simulink model "sgMdl_ModbusRTU_1CLI3SRV"  (R2024b)
settings: Solver=FixedStepAuto  StartTime=0.0  StopTime=inf  RelTol=1e-3  EnableMultiTasking=on
undefined symbols (not defined in the file): standard
libraries: speedgoatlib_mbrtu x14, slrealtimeutilitieslib x10, speedgoatlib_serial x1
Description:
  | Modbus RTU Multi-Node Loopback
settings Model: sg_rtwmakecfg_data=_sg_IO75X_v1_2_0__sg_netxLib_MSVC140_  ModifiedByFormat=Speedgoat  SimulationMode=external  ExtModeTrigDuration=100000  Creator=Speedgoat  LastModifiedBy=Speedgoat
settings SolverCC: ConcurrentTasks=on  AlgebraicLoopSolver=TrustRegion  PositivePriorityOrder=on  AutoInsertRateTranBlk=on  InsertRTBMode=Never (minimum delay)
settings DataIOCC: LimitDataPoints=on  SaveFormat=StructureWithTime  ReturnWorkspaceOutputs=off
settings OptimizationCC: BlockReduction=off  BooleanDataType=off  OptimizeBlockIOStorage=off  BufferReuse=off  GlobalBufferReuse=off  ExpressionFolding=off  LocalBlockOutputs=off  OptimizeDataStoreBuffers=off  BusAssignmentInplaceUpdate=off
settings DebuggingCC: SaveWithParameterizedLinksMsg=none  UnderspecifiedInitializationDetection=Classic  MergeDetectMultiDrivingBlocksExec=none  SignalResolutionControl=TryResolveAllWithWarning  InheritedTsInSrcMsg=none  TasksWithSamePriorityMsg=none  ParameterOverflowMsg=warning  UnconnectedInputMsg=warning  UnconnectedOutputMsg=warning  UnconnectedLineMsg=warning  SFUnexpectedBacktrackingDiag=warning  SFNoUnconditionalDefaultTransitionDiag=warning  SFExecutionAtInitializationDiag=none  ArithmeticOperatorsInVariantConditions=warning
settings HardwareCC: ProdBitPerLong=64  ProdLongLongMode=on  ProdHWDeviceType=Intel->x86-64 (Linux 64)  TargetBitPerPointer=64  TargetBitPerSizeT=64  TargetBitPerPtrDiffT=64  TargetLongLongMode=on  TargetIntDivRoundTo=Zero  TargetEndianess=LittleEndian  TargetWordSize=64  TargetHWDeviceType=MATLAB Host
settings ModelReferenceCC: EnableRefExpFcnMdlSchedulingChecks=on  PropagateSignalLabelsOutOfModel=off
settings SFSimCC: SimUseLocalCustomCode=off  CustomCodeUndefinedFunction=UseInterfaceOnly
settings RTWCC: Description=Speedgoat Real-Time Target Machine  SystemTargetFile=speedgoat.tlc  TemplateMakefile=slrealtime_default_tmf  RetainRTWFile=on  RTWUseLocalCustomCode=off  Toolchain=Simulink Real-Time Toolchain  BuildConfiguration=Faster Runs  TargetLang=C++  GPUComputeCapability=3.5  DLArmComputeVersion=19.05
settings CodeAppCC: StateflowObjectComments=on
settings SimulinkRealTimeTargetCC: SubcomponentCodeInterfacePackaging=Reusable function  InstructionSetFMA=off  LogToMDFFile=off  SLRTFileLogMaxRuns=10
settings ConfigComp: CovMetricSettings=dw  CovSaveCumulativeToWorkspaceVar=on  CovSaveSingleToWorkspaceVar=on  CovExternalEMLEnable=off  CovBoundaryAbsTol=1.0e-5

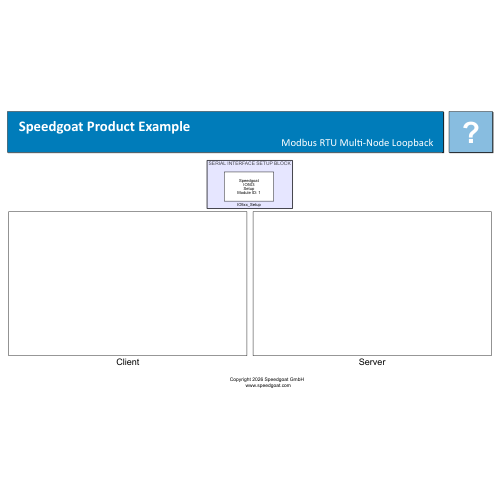
[thumbnail: Simulink's stored preview of the top-level diagram]
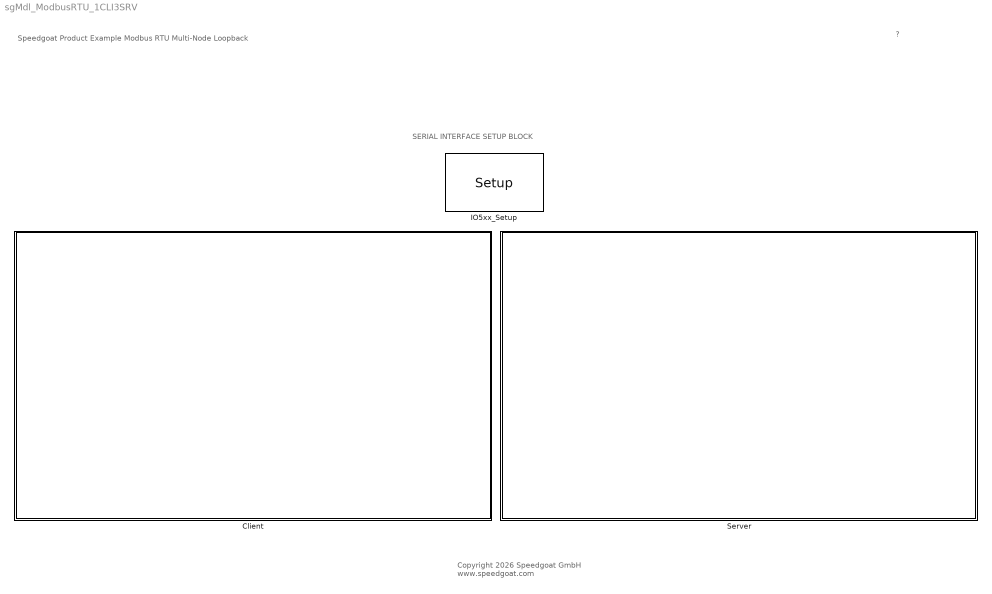
== system sgMdl_ModbusRTU_1CLI3SRV ==
  note: SERIAL INTERFACE SETUP BLOCK
  note: Speedgoat Product Example
      | Modbus RTU Multi-Node Loopback
  note: ?
  note: Copyright 2026 Speedgoat GmbH
      |  www.speedgoat.com
  Client : Subsystem
  IO5xx_Setup : speedgoatlib_serial/Speedgoat Shared blocks/Setup   parModuleType=IO504  parModuleId=1  parSlot=-1  parOscillator=50  parOscillator581=125  parTransceiver1=RS485 Half-Duplex  parTransceiver2=Disabled  parTransceiver3=RS485 Half-Duplex  parTransceiver4=Disabled  parTransceiver5=Disabled  parTransceiver6=Disabled  parTransceiver7=Disabled  parTransceiver8=Disabled  parTxTerm1=on  parRxTerm1=off  parMessageMonitoring1=off  parAutoTurnaround1=off  parTurnaroundDelay1=0  parStandardBaud1=off  parBaudrate1=19200  parBaudDivisor1=25  parSamplingRate1=16x (standard)  parPrescale1=4x  parCalcBaud1=31250  parParity1=Even  parDataBits1=8  parStopBits1=1  parTxTrigLvl1=1  parRxTrigLvl1=56  parHandshake1=none  parRtsHysteresis1=0  parXon1=17  parXoff1=19  parTxSwFifoSize1=1024  parRxSwFifoSize1=1024  parTxTerm2=on  parRxTerm2=off  parMessageMonitoring2=off  parAutoTurnaround2=off  parTurnaroundDelay2=0  parStandardBaud2=off  parBaudrate2=19200  parBaudDivisor2=1  parSamplingRate2=16x (standard)  parPrescale2=None  parCalcBaud2=3125000  parParity2=Even  parDataBits2=8  parStopBits2=1  parTxTrigLvl2=1  parRxTrigLvl2=56  parHandshake2=none  parRtsHysteresis2=0  parXon2=17  parXoff2=19  parTxSwFifoSize2=1024  parRxSwFifoSize2=1024  parTxTerm3=on  parRxTerm3=off  parMessageMonitoring3=off  parAutoTurnaround3=off  parTurnaroundDelay3=0  parStandardBaud3=off  parBaudrate3=19200  parBaudDivisor3=25  parSamplingRate3=16x (standard)  parPrescale3=4x  parCalcBaud3=31250  parParity3=Even  parDataBits3=8  parStopBits3=1  parTxTrigLvl3=1  parRxTrigLvl3=56  parHandshake3=none  parRtsHysteresis3=0  parXon3=17  parXoff3=19  parTxSwFifoSize3=1024  parRxSwFifoSize3=1024  parTxTerm4=off  parRxTerm4=off  parMessageMonitoring4=off  parAutoTurnaround4=off  parTurnaroundDelay4=0  parStandardBaud4=off  parBaudrate4=921600  parBaudDivisor4=1  parSamplingRate4=16x (standard)  parPrescale4=None  parCalcBaud4=3125000  parParity4=None  parDataBits4=8  parStopBits4=1  parTxTrigLvl4=1  parRxTrigLvl4=1  parHandshake4=none  parRtsHysteresis4=0  parXon4=17  parXoff4=19  parTxSwFifoSize4=1024  parRxSwFifoSize4=1024  parTxTerm5=off  parRxTerm5=off  parMessageMonitoring5=off  parAutoTurnaround5=off  parTurnaroundDelay5=0  parStandardBaud5=off  parBaudrate5=921600  parBaudDivisor5=1  parSamplingRate5=16x (standard)  parPrescale5=None  parCalcBaud5=3125000  parParity5=None  parDataBits5=8  parStopBits5=1  parTxTrigLvl5=1  parRxTrigLvl5=1  parHandshake5=none  parRtsHysteresis5=0  parXon5=17  parXoff5=19  parTxSwFifoSize5=1024  parRxSwFifoSize5=1024  parTxTerm6=on  parRxTerm6=off  parMessageMonitoring6=off  parAutoTurnaround6=off  parTurnaroundDelay6=0  parStandardBaud6=off  parBaudrate6=921600  parBaudDivisor6=1  parSamplingRate6=16x (standard)  parPrescale6=None  parCalcBaud6=3125000  parParity6=None  parDataBits6=8  parStopBits6=1  parTxTrigLvl6=1  parRxTrigLvl6=1  parHandshake6=none  parRtsHysteresis6=0  parXon6=17  parXoff6=19  parTxSwFifoSize6=1024  parRxSwFifoSize6=1024  parTxTerm7=off  parRxTerm7=off  parMessageMonitoring7=off  parAutoTurnaround7=off  parTurnaroundDelay7=0  parStandardBaud7=off  parBaudrate7=921600  parBaudDivisor7=1  parSamplingRate7=16x (standard)  parPrescale7=None  parCalcBaud7=3125000  parParity7=None  parDataBits7=8  parStopBits7=1  parTxTrigLvl7=1  parRxTrigLvl7=1  parHandshake7=none  parRtsHysteresis7=0  parXon7=17  parXoff7=19  parTxSwFifoSize7=1024  parRxSwFifoSize7=1024  parTxTerm8=off  parRxTerm8=off  parMessageMonitoring8=off  parAutoTurnaround8=off  parTurnaroundDelay8=0  parStandardBaud8=off  parBaudrate8=921600  parBaudDivisor8=1  parSamplingRate8=16x (standard)  parPrescale8=None  parCalcBaud8=3125000  parParity8=None  parDataBits8=8  parStopBits8=1  parTxTrigLvl8=1  parRxTrigLvl8=1  parHandshake8=none  parRtsHysteresis8=0  parXon8=17  parXoff8=19  parTxSwFifoSize8=1024  parRxSwFifoSize8=1024
  Server : Subsystem

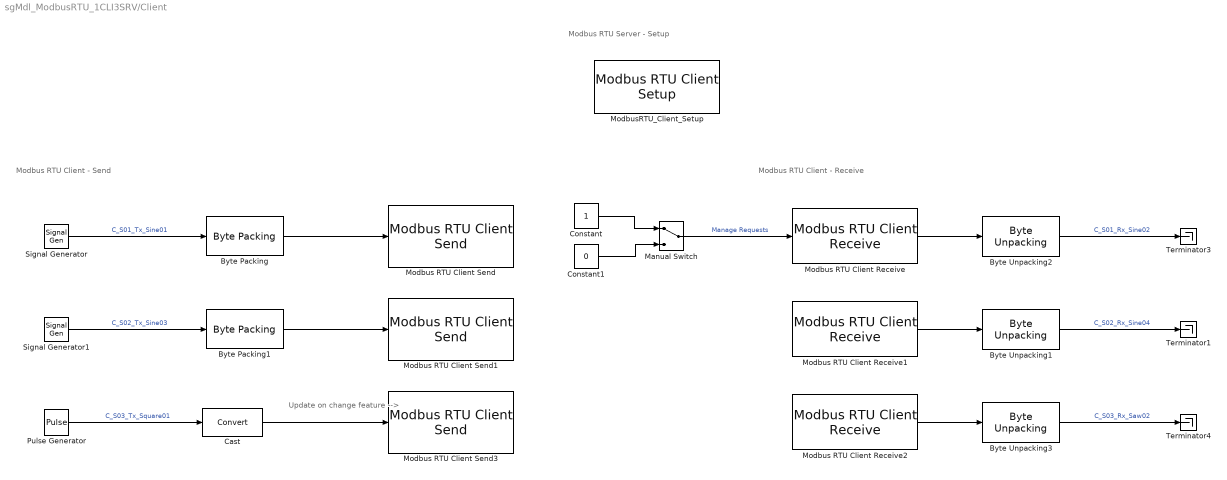
== system sgMdl_ModbusRTU_1CLI3SRV/Client ==
  note: Update on change feature
      | 					-->
  note: Modbus RTU Server - Setup
  note: Modbus RTU Client - Send
  note: Modbus RTU Client - Receive
  Byte Packing : slrealtimeutilitieslib/Byte Packing  MaskPackedDataType=uint16  MaskUnpackedDataTypes={'double'}  MaskAlignment=1
  Byte Packing1 : slrealtimeutilitieslib/Byte Packing  MaskPackedDataType=uint16  MaskUnpackedDataTypes={'double'}  MaskAlignment=1
  Byte Unpacking1 : slrealtimeutilitieslib/Byte Unpacking  MaskUnpackedDataTypes={'double'}  MaskUnpackedDataSizes={[1]}  MaskAlignment=1
  Byte Unpacking2 : slrealtimeutilitieslib/Byte Unpacking  MaskUnpackedDataTypes={'double'}  MaskUnpackedDataSizes={[1]}  MaskAlignment=1
  Byte Unpacking3 : slrealtimeutilitieslib/Byte Unpacking  MaskUnpackedDataTypes={'double'}  MaskUnpackedDataSizes={[1]}  MaskAlignment=1
  Cast : DataTypeConversion  SaturateOnIntegerOverflow=off  RndMeth=Floor
  Constant : Constant  OutDataTypeStr=boolean
  Constant1 : Constant  Value=0  OutDataTypeStr=boolean
  Manual Switch : ManualSwitch
  Modbus RTU Client Receive : speedgoatlib_mbrtu/Client/Modbus RTU Client Receive  InterfaceID=1211  NodeID=1  FunctionCode=FC4 (Read Multiple Input Registers)  DataIndex=0  DataQuantity=4  ByteSwap=off  PollingIntervall=1000  ManageRequest=on  SampleTime=-1  UpdateChange=off
      settings: SourceProductName=Modbus RTU
      settings: AttributesFormatString=|
      | %<FunctionCode>
      | Server Node: %<NodeID> | Address Index: %<DataIndex> | Quantity: %<DataQuantity>
  Modbus RTU Client Receive1 : speedgoatlib_mbrtu/Client/Modbus RTU Client Receive  InterfaceID=1211  NodeID=2  FunctionCode=FC4 (Read Multiple Input Registers)  DataIndex=10  DataQuantity=4  ByteSwap=off  PollingIntervall=500  ManageRequest=off  SampleTime=-1  UpdateChange=off
      settings: SourceProductName=Modbus RTU
      settings: AttributesFormatString=|
      | %<FunctionCode>
      | Server Node: %<NodeID> | Address Index: %<DataIndex> | Quantity: %<DataQuantity>
  Modbus RTU Client Receive2 : speedgoatlib_mbrtu/Client/Modbus RTU Client Receive  InterfaceID=1211  NodeID=3  FunctionCode=FC4 (Read Multiple Input Registers)  DataIndex=0  DataQuantity=4  ByteSwap=off  PollingIntervall=500  ManageRequest=off  SampleTime=-1  UpdateChange=off
      settings: SourceProductName=Modbus RTU
      settings: AttributesFormatString=|
      | %<FunctionCode>
      | Server Node: %<NodeID> | Address Index: %<DataIndex> | Quantity: %<DataQuantity>
  Modbus RTU Client Send : speedgoatlib_mbrtu/Client/Modbus RTU Client Send  InterfaceID=1211  NodeID=1  FunctionCode=FC16 (Write Multiple Holding Registers)  DataIndex=0  DataQuantity=4  ByteSwap=off  PollingIntervall=1000  ManageRequest=off  SampleTime=-1  UpdateChange=off
      settings: SourceProductName=Modbus RTU
      settings: AttributesFormatString=|
      | %<FunctionCode>
      | Server Node: %<NodeID> | Address Index: %<DataIndex> | Quantity: %<DataQuantity>
  Modbus RTU Client Send1 : speedgoatlib_mbrtu/Client/Modbus RTU Client Send  InterfaceID=1211  NodeID=2  FunctionCode=FC16 (Write Multiple Holding Registers)  DataIndex=4  DataQuantity=4  ByteSwap=off  PollingIntervall=500  ManageRequest=off  SampleTime=-1  UpdateChange=off
      settings: SourceProductName=Modbus RTU
      settings: AttributesFormatString=|
      | %<FunctionCode>
      | Server Node: %<NodeID> | Address Index: %<DataIndex> | Quantity: %<DataQuantity>
  Modbus RTU Client Send3 : speedgoatlib_mbrtu/Client/Modbus RTU Client Send  InterfaceID=1211  NodeID=3  FunctionCode=FC6 (Write Single Holding Register)  DataIndex=5  DataQuantity=1  ByteSwap=off  PollingIntervall=500  ManageRequest=off  SampleTime=-1  UpdateChange=off
      settings: SourceProductName=Modbus RTU
      settings: AttributesFormatString=|
      | %<FunctionCode>
      | Server Node: %<NodeID> | Address Index: %<DataIndex> | Quantity: %<DataQuantity>
  "ModbusRTU_Client_Setup " : speedgoatlib_mbrtu/Client/Modbus RTU Client Setup  SerialInterface=IO504  InterfaceModuleID=1  SerialPort=1  InterfaceID=1211  AutoID=on  RespDelay=10  ByteSwap=off  Successive=off  SampleTime=-1
      settings: AttributesFormatString=Interface: %<SerialInterface> | Channel: %<SerialPort>  SourceProductName=Modbus RTU
  Pulse Generator : DiscretePulseGenerator  PulseType=Time based  Amplitude=55  Period=5  PulseWidth=65  PhaseDelay=1
  Signal Generator : SignalGenerator  Amplitude=10  Frequency=0.1  Units=rad/sec
  Signal Generator1 : SignalGenerator  Amplitude=30  Frequency=0.3  Units=rad/sec
  Terminator1 : Terminator
  Terminator3 : Terminator
  Terminator4 : Terminator
  wires:
  Manual Switch/1 -> Modbus RTU Client Receive/1  "Manage Requests"
  Constant1/1 -> Manual Switch/2
  Byte Packing/1 -> Modbus RTU Client Send/1
  Modbus RTU Client Receive1/1 -> Byte Unpacking1/1
  Pulse Generator/1 -> Cast/1  "C_S03_Tx_Square01"
  Modbus RTU Client Receive2/1 -> Byte Unpacking3/1
  Byte Packing1/1 -> Modbus RTU Client Send1/1
  Modbus RTU Client Receive/1 -> Byte Unpacking2/1
  Signal Generator/1 -> Byte Packing/1  "C_S01_Tx_Sine01"
  Constant/1 -> Manual Switch/1
  Byte Unpacking2/1 -> Terminator3/1  "C_S01_Rx_Sine02"
  Signal Generator1/1 -> Byte Packing1/1  "C_S02_Tx_Sine03"
  Byte Unpacking1/1 -> Terminator1/1  "C_S02_Rx_Sine04"
  Byte Unpacking3/1 -> Terminator4/1  "C_S03_Rx_Saw02"
  Cast/1 -> Modbus RTU Client Send3/1

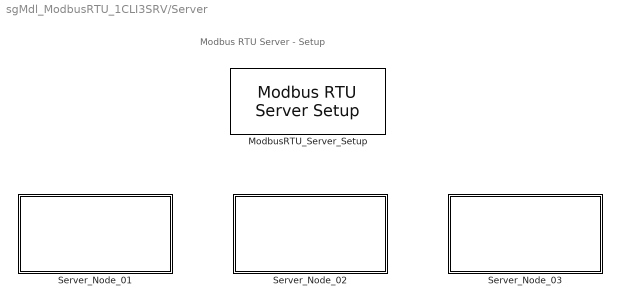
== system sgMdl_ModbusRTU_1CLI3SRV/Server ==
  note: Modbus RTU Server - Setup
  "ModbusRTU_Server_Setup " : speedgoatlib_mbrtu/Server/Modbus RTU Server Setup  SerialInterface=IO504  InterfaceModuleID=1  SerialPort=3  InterfaceID=2213  AutoID=on  Nodes=[1,2,3]  TableDim=[255,255,255,255;100,100,100,100;64,64,64,64]  RespDelay=0  Swap=off  SampleTime=-1
      settings: AttributesFormatString=Interface: %<SerialInterface> | Channel: %<SerialPort>  SourceProductName=Modbus RTU
  Server_Node_01 : Subsystem
  Server_Node_02 : Subsystem
  Server_Node_03 : Subsystem

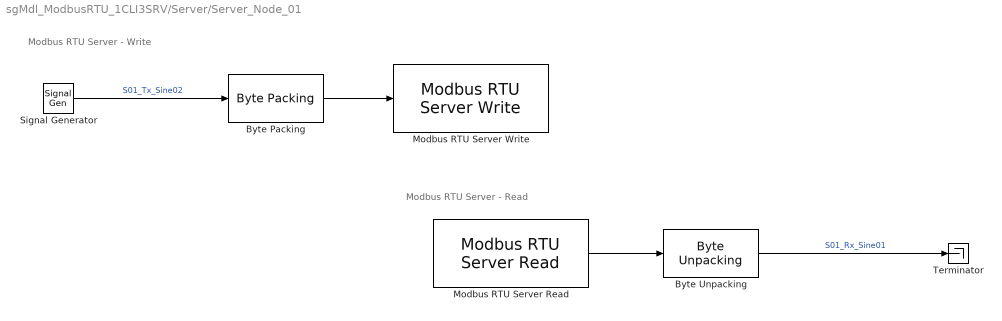
== system sgMdl_ModbusRTU_1CLI3SRV/Server/Server_Node_01 ==
  note: Modbus RTU Server - Read
  note: Modbus RTU Server - Write
  Byte Packing : slrealtimeutilitieslib/Byte Packing  MaskPackedDataType=uint16  MaskUnpackedDataTypes={'double'}  MaskAlignment=1
  Byte Unpacking : slrealtimeutilitieslib/Byte Unpacking  MaskUnpackedDataTypes={'double'}  MaskUnpackedDataSizes={[1]}  MaskAlignment=1
  Modbus RTU Server Read : speedgoatlib_mbrtu/Server/Modbus RTU Server Read  ServerID=2213  NodeID=1  DataTable=Holding Registers  DataIndex=0  DataQuantity=4  ByteSwap=off  SampleTime=-1
      settings: AttributesFormatString=%<DataTable> - Index: %<DataIndex> - Quantity: %<DataQuantity>  SourceProductName=Modbus RTU
  Modbus RTU Server Write : speedgoatlib_mbrtu/Server/Modbus RTU Server Write  ServerID=2213  NodeID=1  DataTable=Input Registers  DataIndex=0  DataQuantity=4  ByteSwap=off  SampleTime=-1
      settings: AttributesFormatString=%<DataTable> - Index: %<DataIndex> - Quantity: %<DataQuantity>  SourceProductName=Modbus RTU
  Signal Generator : SignalGenerator  Amplitude=40  Frequency=0.4  Units=rad/sec
  Terminator : Terminator
  wires:
  Signal Generator/1 -> Byte Packing/1  "S01_Tx_Sine02"
  Byte Packing/1 -> Modbus RTU Server Write/1
  Byte Unpacking/1 -> Terminator/1  "S01_Rx_Sine01"
  Modbus RTU Server Read/1 -> Byte Unpacking/1

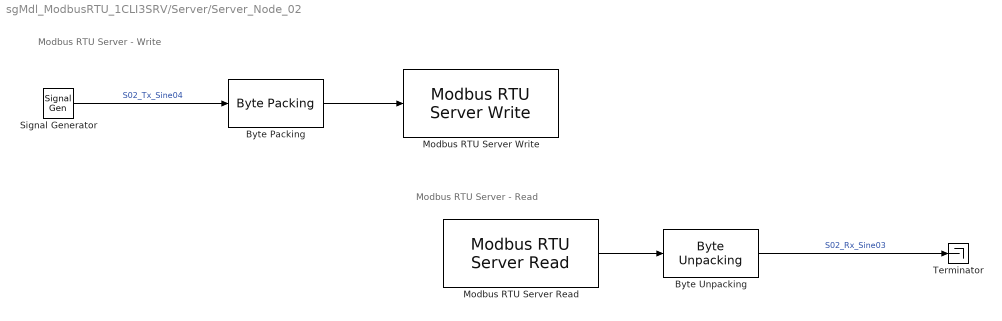
== system sgMdl_ModbusRTU_1CLI3SRV/Server/Server_Node_02 ==
  note: Modbus RTU Server - Read
  note: Modbus RTU Server - Write
  Byte Packing : slrealtimeutilitieslib/Byte Packing  MaskPackedDataType=uint16  MaskUnpackedDataTypes={'double'}  MaskAlignment=1
  Byte Unpacking : slrealtimeutilitieslib/Byte Unpacking  MaskUnpackedDataTypes={'double'}  MaskUnpackedDataSizes={[1]}  MaskAlignment=1
  Modbus RTU Server Read : speedgoatlib_mbrtu/Server/Modbus RTU Server Read  ServerID=2213  NodeID=2  DataTable=Holding Registers  DataIndex=4  DataQuantity=4  ByteSwap=off  SampleTime=-1
      settings: AttributesFormatString=%<DataTable> - Index: %<DataIndex> - Quantity: %<DataQuantity>  SourceProductName=Modbus RTU
  Modbus RTU Server Write : speedgoatlib_mbrtu/Server/Modbus RTU Server Write  ServerID=2213  NodeID=2  DataTable=Input Registers  DataIndex=10  DataQuantity=4  ByteSwap=off  SampleTime=-1
      settings: AttributesFormatString=%<DataTable> - Index: %<DataIndex> - Quantity: %<DataQuantity>  SourceProductName=Modbus RTU
  Signal Generator : SignalGenerator  Amplitude=80  Frequency=0.8  Units=rad/sec
  Terminator : Terminator
  wires:
  Modbus RTU Server Read/1 -> Byte Unpacking/1
  Byte Unpacking/1 -> Terminator/1  "S02_Rx_Sine03"
  Byte Packing/1 -> Modbus RTU Server Write/1
  Signal Generator/1 -> Byte Packing/1  "S02_Tx_Sine04"

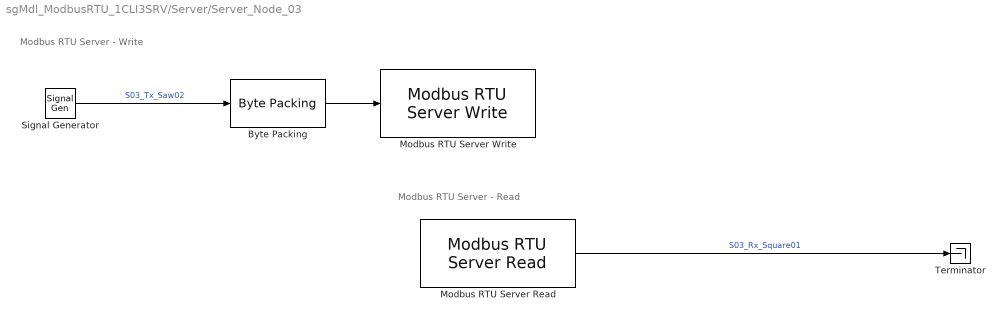
== system sgMdl_ModbusRTU_1CLI3SRV/Server/Server_Node_03 ==
  note: Modbus RTU Server - Write
  note: Modbus RTU Server - Read
  Byte Packing : slrealtimeutilitieslib/Byte Packing  MaskPackedDataType=uint16  MaskUnpackedDataTypes={'double'}  MaskAlignment=1
  Modbus RTU Server Read : speedgoatlib_mbrtu/Server/Modbus RTU Server Read  ServerID=2213  NodeID=3  DataTable=Holding Registers  DataIndex=5  DataQuantity=1  ByteSwap=off  SampleTime=-1
      settings: AttributesFormatString=%<DataTable> - Index: %<DataIndex> - Quantity: %<DataQuantity>  SourceProductName=Modbus RTU
  Modbus RTU Server Write : speedgoatlib_mbrtu/Server/Modbus RTU Server Write  ServerID=2213  NodeID=3  DataTable=Input Registers  DataIndex=0  DataQuantity=4  ByteSwap=off  SampleTime=-1
      settings: AttributesFormatString=%<DataTable> - Index: %<DataIndex> - Quantity: %<DataQuantity>  SourceProductName=Modbus RTU
  Signal Generator : SignalGenerator  WaveForm=sawtooth  Amplitude=20  Frequency=0.2  Units=rad/sec
  Terminator : Terminator
  wires:
  Modbus RTU Server Read/1 -> Terminator/1  "S03_Rx_Square01"
  Byte Packing/1 -> Modbus RTU Server Write/1
  Signal Generator/1 -> Byte Packing/1  "S03_Tx_Saw02"
